simulink model "CrazyClover_trajectory_tracking"  (R2020b)
settings: Solver=VariableStepAuto  StartTime=0.0  StopTime=30  RelTol=1e-3
values from neighbouring files (symbols this model uses):
  controller_matrix = [mass/(4*gravity)*1000 mass/(4*gravity)*1000 mass/(4*gravity)*1000 mass/(4*gravity)*1000 ... (first row only)    [sim_param.m]
  kM1 = Armlength /sqrt(2)    [sim_param.m]
  kM2 = Armlength /sqrt(2)    [sim_param.m]
  kM3 = 1    [sim_param.m]
undefined symbols (not defined in the file or in its folder): Pitchrate, Rollrate, traj, Yawrate
libraries: pid_lib x6
settings Model: Creator=kt012  LastModifiedBy=kt012

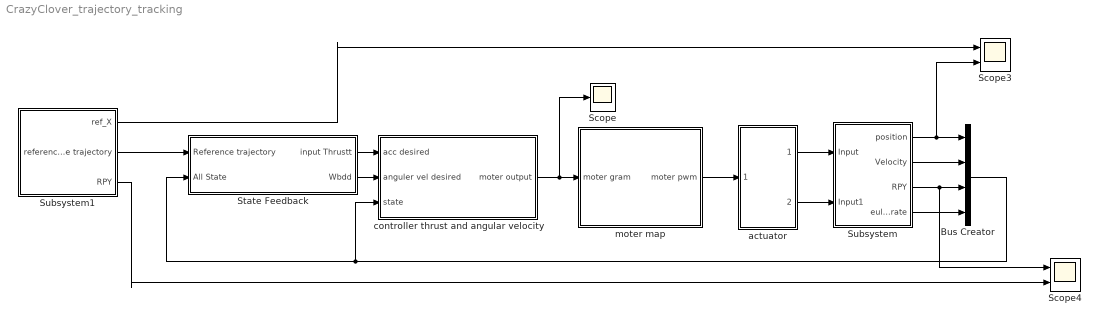
== system CrazyClover_trajectory_tracking ==
  Bus Creator : BusCreator  Inputs=4
  Scope : Scope
  Scope3 : Scope  NumInputPorts=2
  Scope4 : Scope  NumInputPorts=2
  State Feedback : Subsystem
  Subsystem : Subsystem
  Subsystem1 : Subsystem
  actuator : Subsystem
  controller thrust and angular velocity : Subsystem
  moter map : Subsystem
  wires:
  actuator/1(Input) -> Subsystem/1(Input)
  State Feedback/2("Wbdd ") -> controller thrust and angular velocity/2(anguler vel desired)
  actuator/2(Input1) -> Subsystem/2(Input1)
  Subsystem/1(position) -> Scope3/2, Bus Creator/1
  controller thrust and angular velocity/1(moter output) -> Scope/1, moter map/1(moter gram)
  State Feedback/1(input Thrustt) -> controller thrust and angular velocity/1(acc desired)
  moter map/1(moter pwm) -> actuator/1(PWM)
  Subsystem/3(RPY) -> Scope4/1, Bus Creator/3
  Subsystem/4(euler rate) -> Bus Creator/4
  Subsystem/2(Velocity) -> Bus Creator/2
  Bus Creator/1 -> controller thrust and angular velocity/3(state), State Feedback/2(All State)
  Subsystem1/1(ref_X) -> Scope3/1
  Subsystem1/2(reference trajectory) -> State Feedback/1(Reference trajectory)
  Subsystem1/3(RPY) -> Scope4/2

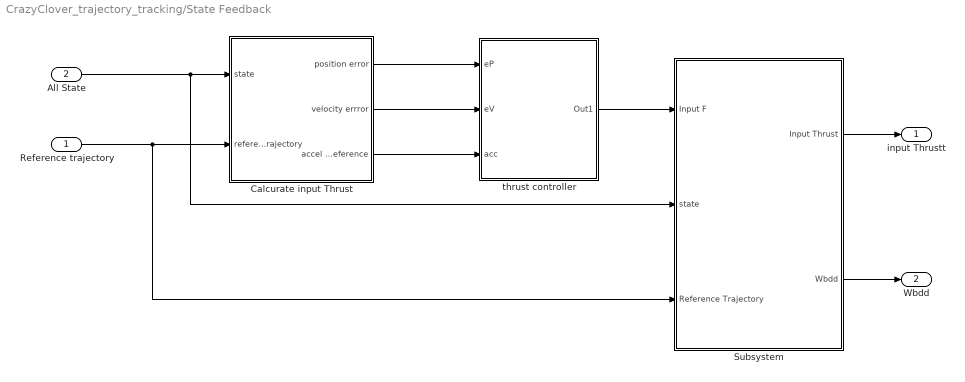
== system CrazyClover_trajectory_tracking/State Feedback ==
  Reference trajectory : Inport
  All State : Inport  Port=2
  Calcurate input Thrust : Subsystem
  Subsystem : Subsystem
  thrust controller : Subsystem
  input Thrustt : Outport
  "Wbdd " : Outport  Port=2  VectorParamsAs1DForOutWhenUnconnected=off
  wires:
  All State/1 -> Calcurate input Thrust/1(state), Subsystem/2(state)
  Reference trajectory/1 -> Calcurate input Thrust/2(reference trajectory), Subsystem/3(Reference Trajectory)
  Subsystem/2("Wbdd ") -> "Wbdd "/1
  Subsystem/1(Input Thrust) -> input Thrustt/1
  Calcurate input Thrust/1(position error) -> thrust controller/1(eP)
  Calcurate input Thrust/2(velocity errror) -> thrust controller/2(eV)
  Calcurate input Thrust/3(accel reference) -> thrust controller/3(acc)
  thrust controller/1(Out1) -> Subsystem/1(Input F)

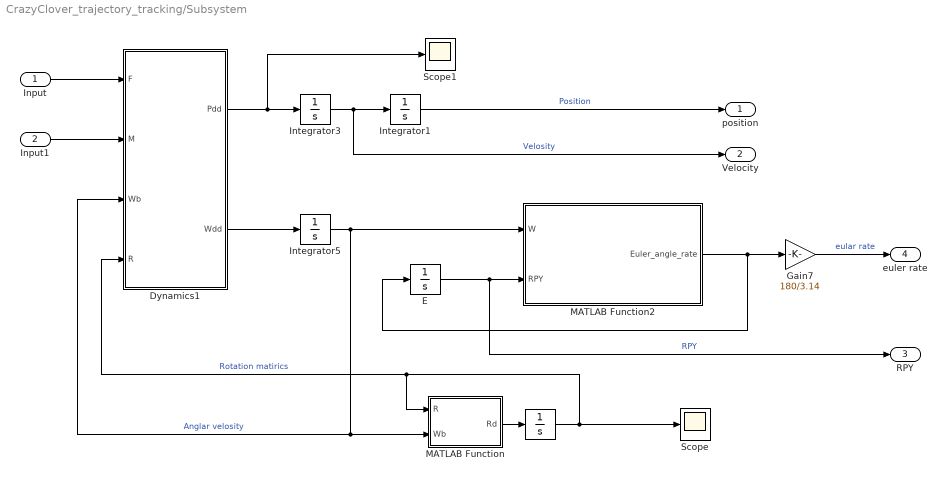
== system CrazyClover_trajectory_tracking/Subsystem ==
  Input : Inport
  Input1 : Inport  Port=2
  " " : Integrator  InitialCondition=[1 0 0; 0 1 0; 0 0 1];  ContinuousStateAttributes="\"\""
  Dynamics1 : MATLAB Function  TreatAsAtomicUnit=on
  E : Integrator  InitialCondition=[0 0 0];
  Gain7 : Gain  Gain=180/3.14
  Integrator1 : Integrator  InitialCondition=[0 0 0];
  Integrator3 : Integrator  InitialCondition=[0 0 0];
  Integrator5 : Integrator  InitialCondition=[0 0 0];
  MATLAB Function : MATLAB Function  TreatAsAtomicUnit=on
  MATLAB Function2 : MATLAB Function  TreatAsAtomicUnit=on
  Scope : Scope
  Scope1 : Scope
  position : Outport
  Velocity : Outport  Port=2
  RPY : Outport  Port=3
  euler rate : Outport  Port=4
  wires:
  MATLAB Function2/1(Euler_angle_rate) -> E/1, Gain7/1
  Dynamics1/1(Pdd) -> Integrator3/1, Scope1/1
  Integrator1/1 -> position/1  "Position"
  Integrator3/1 -> Velocity/1, Integrator1/1  "Velosity"
  E/1 -> RPY/1, MATLAB Function2/2(RPY)  "RPY"
  Dynamics1/2(Wdd) -> Integrator5/1
  Gain7/1 -> euler rate/1  "eular rate"
  MATLAB Function/1(Rd) -> " "/1
  Integrator5/1 -> MATLAB Function/2(Wb), Dynamics1/3(Wb), MATLAB Function2/1(W)  "Anglar velosity"
  " "/1 -> Dynamics1/4(R), MATLAB Function/1(R), Scope/1  "Rotation matirics"
  Input1/1 -> Dynamics1/2(M)
  Input/1 -> Dynamics1/1(F)

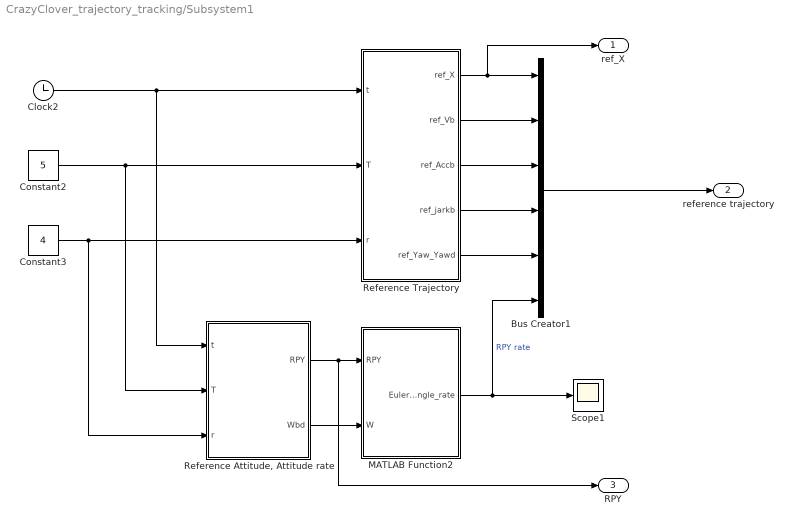
== system CrazyClover_trajectory_tracking/Subsystem1 ==
  Bus Creator1 : BusCreator  Inputs=6
  Clock2 : Clock
  Constant2 : Constant  Value=5
  Constant3 : Constant  Value=4
  MATLAB Function2 : MATLAB Function  TreatAsAtomicUnit=on
  "Reference Attitude, Attitude rate " : MATLAB Function  TreatAsAtomicUnit=on
  Reference Trajectory : MATLAB Function  TreatAsAtomicUnit=on
  Scope1 : Scope
  ref_X : Outport
  reference trajectory : Outport  Port=2
  RPY : Outport  Port=3
  wires:
  Reference Trajectory/1(ref_X) -> ref_X/1, Bus Creator1/1
  Reference Trajectory/4(ref_jarkb) -> Bus Creator1/4
  Reference Trajectory/3(ref_Accb) -> Bus Creator1/3
  MATLAB Function2/1(Euler_angle_rate) -> Bus Creator1/6, Scope1/1  "RPY rate"
  Constant3/1 -> "Reference Attitude, Attitude rate "/3(r), Reference Trajectory/3(r)
  Reference Trajectory/5(ref_Yaw_Yawd) -> Bus Creator1/5
  Clock2/1 -> "Reference Attitude, Attitude rate "/1(t), Reference Trajectory/1(t)
  Constant2/1 -> "Reference Attitude, Attitude rate "/2(T), Reference Trajectory/2(T)
  "Reference Attitude, Attitude rate "/2(Wbd) -> MATLAB Function2/2(W)
  Reference Trajectory/2(ref_Vb) -> Bus Creator1/2
  Bus Creator1/1 -> reference trajectory/1
  "Reference Attitude, Attitude rate "/1(RPY) -> RPY/1, MATLAB Function2/1(RPY)

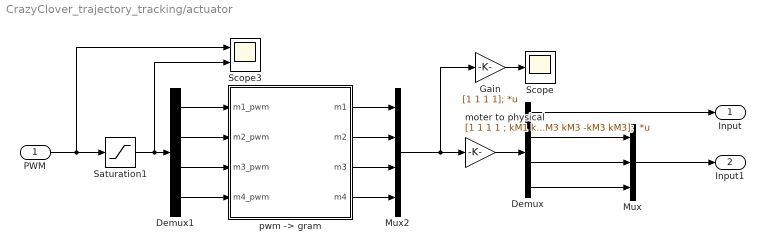
== system CrazyClover_trajectory_tracking/actuator ==
  PWM : Inport
  Demux : Demux
  Demux1 : Demux
  Gain : Gain  Gain=[1 1 1 1];  Multiplication=Matrix(K*u)
  Mux : Mux  Inputs=3
  Mux2 : Mux
  Saturation1 : Saturate  UpperLimit=40000  LowerLimit=0
  Scope : Scope
  Scope3 : Scope  NumInputPorts=2
  moter to physical : Gain  Gain=[1 1 1 1 ; kM1 kM1 -kM1 -kM1; -kM2 kM2 kM2 -kM2; -kM3 kM3 -kM3 kM3];  Multiplication=Matrix(K*u)
  "pwm -> gram" : MATLAB Function  TreatAsAtomicUnit=on
  Input : Outport
  Input1 : Outport  Port=2
  wires:
  Demux/2 -> Mux/1
  "pwm -> gram"/3(m3) -> Mux2/3
  Demux1/2 -> "pwm -> gram"/2(m2_pwm)
  Demux/4 -> Mux/3
  Demux/3 -> Mux/2
  moter to physical/1 -> Demux/1
  "pwm -> gram"/1(m1) -> Mux2/1
  Mux2/1 -> Gain/1, moter to physical/1
  Gain/1 -> Scope/1
  Saturation1/1 -> Scope3/2, Demux1/1
  PWM/1 -> Scope3/1, Saturation1/1
  Demux1/3 -> "pwm -> gram"/3(m3_pwm)
  "pwm -> gram"/4(m4) -> Mux2/4
  "pwm -> gram"/2(m2) -> Mux2/2
  Demux1/4 -> "pwm -> gram"/4(m4_pwm)
  Demux1/1 -> "pwm -> gram"/1(m1_pwm)
  Mux/1 -> Input1/1
  Demux/1 -> Input/1

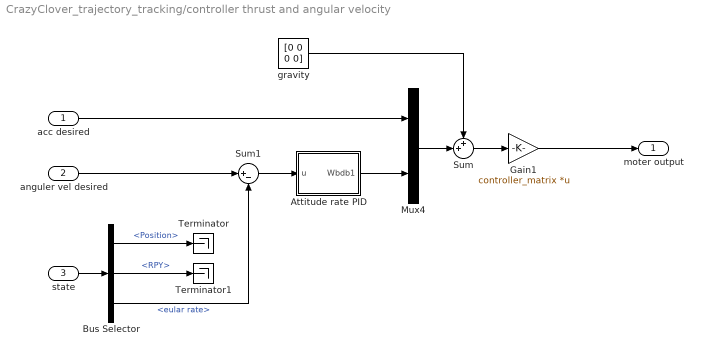
== system CrazyClover_trajectory_tracking/controller thrust and angular velocity ==
  acc desired : Inport
  anguler vel desired : Inport  Port=2
  state : Inport  Port=3
  Attitude rate PID : Subsystem
  Bus Selector : BusSelector  OutputSignals=Position,RPY,eular rate
  Gain1 : Gain  Gain=controller_matrix  Multiplication=Matrix(K*u)
  Mux4 : Mux  Inputs=2
  Sum : Sum  Inputs=++|
  Sum1 : Sum  Inputs=|+-
  Terminator : Terminator
  Terminator1 : Terminator
  gravity : Constant  Value=[0 0 0 0]
  moter output : Outport
  wires:
  Sum/1 -> Gain1/1
  Gain1/1 -> moter output/1
  Mux4/1 -> Sum/2
  gravity/1 -> Sum/1
  Attitude rate PID/1(Wbdb1) -> Mux4/2
  state/1 -> Bus Selector/1
  Bus Selector/3 -> Sum1/2  "<eular rate>"
  Sum1/1 -> Attitude rate PID/1(u)
  Bus Selector/1 -> Terminator/1  "<Position>"
  Bus Selector/2 -> Terminator1/1  "<RPY>"
  anguler vel desired/1 -> Sum1/1
  acc desired/1 -> Mux4/1

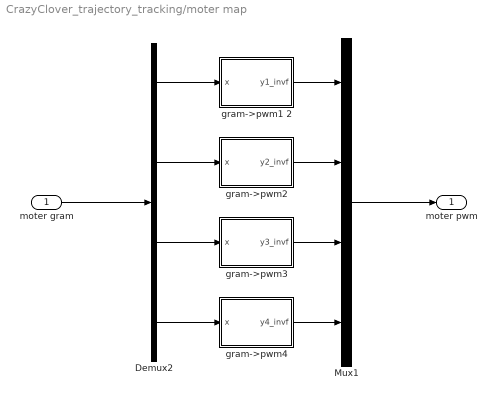
== system CrazyClover_trajectory_tracking/moter map ==
  moter gram : Inport
  Demux2 : Demux
  Mux1 : Mux
  gram->pwm1 2 : MATLAB Function  TreatAsAtomicUnit=on
  gram->pwm2 : MATLAB Function  TreatAsAtomicUnit=on
  gram->pwm3 : MATLAB Function  TreatAsAtomicUnit=on
  gram->pwm4 : MATLAB Function  TreatAsAtomicUnit=on
  moter pwm : Outport
  wires:
  Demux2/4 -> gram->pwm4/1(x)
  Demux2/3 -> gram->pwm3/1(x)
  gram->pwm4/1(y4_invf) -> Mux1/4
  Demux2/2 -> gram->pwm2/1(x)
  gram->pwm3/1(y3_invf) -> Mux1/3
  gram->pwm2/1(y2_invf) -> Mux1/2
  gram->pwm1 2/1(y1_invf) -> Mux1/1
  Demux2/1 -> gram->pwm1 2/1(x)
  Mux1/1 -> moter pwm/1
  moter gram/1 -> Demux2/1

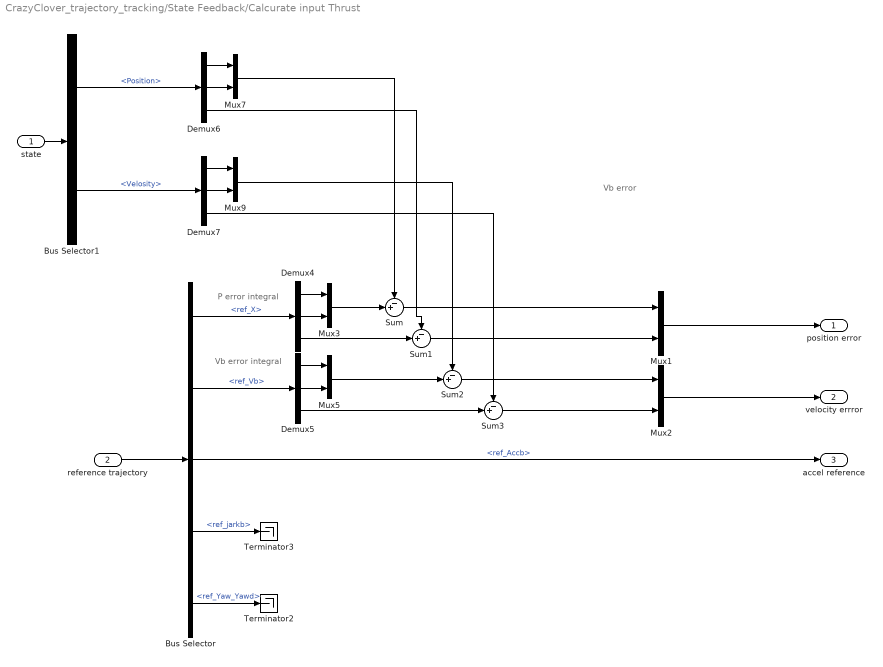
== system CrazyClover_trajectory_tracking/State Feedback/Calcurate input Thrust ==
  note: P error integral
  note: Vb error
  note: Vb error integral
  state : Inport
  reference trajectory : Inport  Port=2
  Bus Selector : BusSelector  OutputSignals=ref_X,ref_Vb,ref_Accb,ref_jarkb,ref_Yaw_Yawd
  Bus Selector1 : BusSelector  OutputSignals=Position,Velosity
  Demux{4..7} (4 alike) : Demux  Outputs=3
  Mux{1..3,5,7,9} (6 alike) : Mux  Inputs=2
  Sum{,1..3} (4 alike) : Sum  Inputs=-+|
  Terminator2 : Terminator
  Terminator3 : Terminator
  position error : Outport
  velocity errror : Outport  Port=2
  accel reference : Outport  Port=3
  wires:
  Demux6/2 -> Mux7/2
  Demux5/3 -> Sum3/2
  Bus Selector/1 -> Demux4/1  "<ref_X>"
  reference trajectory/1 -> Bus Selector/1
  Mux5/1 -> Sum2/2
  Bus Selector/5 -> Terminator2/1  "<ref_Yaw_Yawd>"
  Sum3/1 -> Mux2/2
  Bus Selector/4 -> Terminator3/1  "<ref_jarkb>"
  Mux2/1 -> velocity errror/1
  Demux4/1 -> Mux3/1
  Bus Selector/3 -> accel reference/1  "<ref_Accb>"
  state/1 -> Bus Selector1/1
  Demux4/3 -> Sum1/2
  Sum2/1 -> Mux2/1
  Bus Selector1/1 -> Demux6/1  "<Position>"
  Demux6/1 -> Mux7/1
  Demux7/3 -> Sum3/1
  Mux1/1 -> position error/1
  Mux7/1 -> Sum/1
  Mux9/1 -> Sum2/1
  Sum1/1 -> Mux1/2
  Bus Selector1/2 -> Demux7/1  "<Velosity>"
  Demux4/2 -> Mux3/2
  Demux5/2 -> Mux5/2
  Sum/1 -> Mux1/1
  Demux7/1 -> Mux9/1
  Bus Selector/2 -> Demux5/1  "<ref_Vb>"
  Demux7/2 -> Mux9/2
  Demux6/3 -> Sum1/1
  Demux5/1 -> Mux5/1
  Mux3/1 -> Sum/2

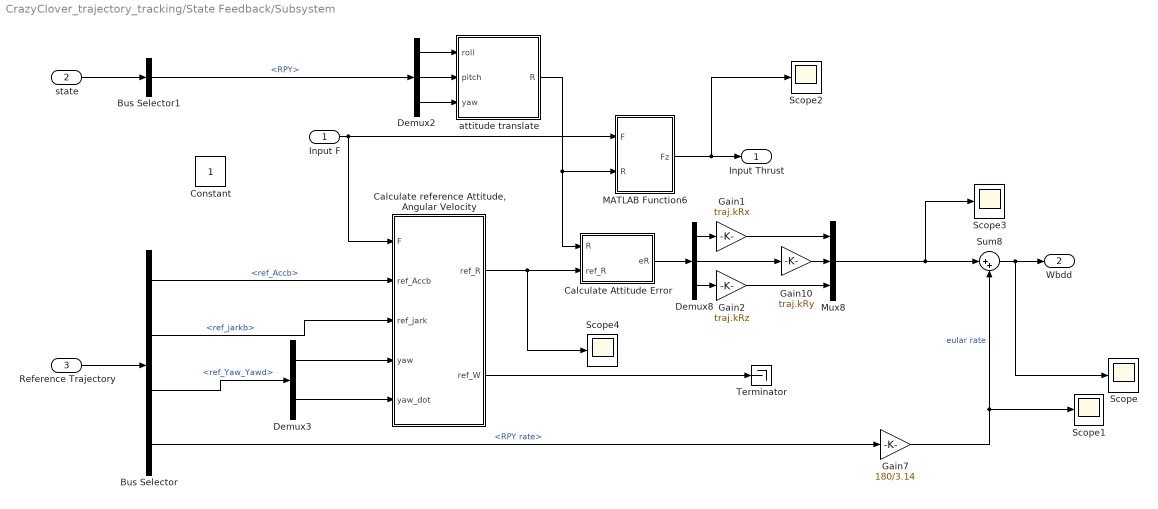
== system CrazyClover_trajectory_tracking/State Feedback/Subsystem ==
  Input F : Inport
  state : Inport  Port=2
  Reference Trajectory : Inport  Port=3
  Bus Selector : BusSelector  OutputSignals=ref_Accb,ref_jarkb,ref_Yaw_Yawd,RPY rate
  Bus Selector1 : BusSelector  OutputSignals=RPY
  Calculate Attitude Error : MATLAB Function  TreatAsAtomicUnit=on
  "Calculate reference Attitude, Angular Velocity" : MATLAB Function  TreatAsAtomicUnit=on
  Constant : Constant
  Demux2 : Demux  Outputs=3
  Demux3 : Demux  Outputs=2
  Demux8 : Demux  Outputs=3
  Gain1 : Gain  Gain=traj.kRx
  Gain10 : Gain  Gain=traj.kRy
  Gain2 : Gain  Gain=traj.kRz
  Gain7 : Gain  Gain=180/3.14
  MATLAB Function6 : MATLAB Function
  Mux8 : Mux  Inputs=3
  Scope{,1..4} (5 alike) : Scope
  Sum8 : Sum  Inputs=|++
  Terminator : Terminator
  attitude translate : MATLAB Function  TreatAsAtomicUnit=on
  Input Thrust : Outport
  "Wbdd " : Outport  Port=2  VectorParamsAs1DForOutWhenUnconnected=off
  wires:
  Demux8/3 -> Gain2/1
  "Calculate reference Attitude, Angular Velocity"/1(ref_R) -> Scope4/1, Calculate Attitude Error/2(ref_R)
  Sum8/1 -> Scope/1, "Wbdd "/1
  Input F/1 -> "Calculate reference Attitude, Angular Velocity"/1(F), MATLAB Function6/1(F)
  Demux8/2 -> Gain10/1
  attitude translate/1(R) -> Calculate Attitude Error/1(R), MATLAB Function6/2(R)
  Demux8/1 -> Gain1/1
  Gain10/1 -> Mux8/2
  Bus Selector1/1 -> Demux2/1  "<RPY>"
  Bus Selector/3 -> Demux3/1  "<ref_Yaw_Yawd>"
  Reference Trajectory/1 -> Bus Selector/1
  Bus Selector/1 -> "Calculate reference Attitude, Angular Velocity"/2(ref_Accb)  "<ref_Accb>"
  Demux3/1 -> "Calculate reference Attitude, Angular Velocity"/4(yaw)
  Demux3/2 -> "Calculate reference Attitude, Angular Velocity"/5(yaw_dot)
  state/1 -> Bus Selector1/1
  MATLAB Function6/1(Fz) -> Scope2/1, Input Thrust/1
  Bus Selector/2 -> "Calculate reference Attitude, Angular Velocity"/3(ref_jark)  "<ref_jarkb>"
  Demux2/1 -> attitude translate/1(roll)
  Demux2/2 -> attitude translate/2(pitch)
  Demux2/3 -> attitude translate/3(yaw)
  Calculate Attitude Error/1(eR) -> Demux8/1
  "Calculate reference Attitude, Angular Velocity"/2(ref_W) -> Terminator/1
  Bus Selector/4 -> Gain7/1  "<RPY rate>"
  Mux8/1 -> Scope3/1, Sum8/1
  Gain1/1 -> Mux8/1
  Gain2/1 -> Mux8/3
  Gain7/1 -> Sum8/2, Scope1/1  "eular rate"

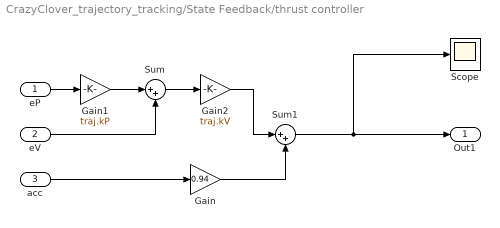
== system CrazyClover_trajectory_tracking/State Feedback/thrust controller ==
  eP : Inport
  eV : Inport  Port=2
  acc : Inport  Port=3
  Gain : Gain  Gain=0.94
  Gain1 : Gain  Gain=traj.kP
  Gain2 : Gain  Gain=traj.kV
  Scope : Scope
  Sum : Sum  Inputs=|++
  Sum1 : Sum  Inputs=|++
  Out1 : Outport
  wires:
  acc/1 -> Gain/1
  Sum/1 -> Gain2/1
  Sum1/1 -> Scope/1, Out1/1
  eP/1 -> Gain1/1
  eV/1 -> Sum/2
  Gain1/1 -> Sum/1
  Gain2/1 -> Sum1/1
  Gain/1 -> Sum1/2

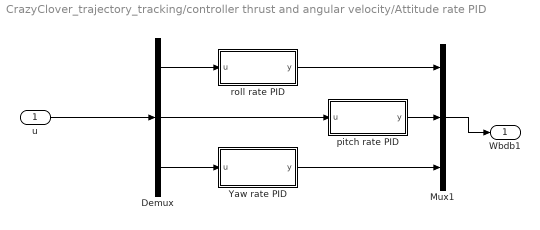
== system CrazyClover_trajectory_tracking/controller thrust and angular velocity/Attitude rate PID ==
  u : Inport
  Demux : Demux  Outputs=3
  Mux1 : Mux  Inputs=3
  "Yaw rate PID " : Subsystem
  pitch rate PID : Subsystem
  "roll rate PID " : Subsystem
  Wbdb1 : Outport
  wires:
  "roll rate PID "/1(y) -> Mux1/1
  pitch rate PID/1(y) -> Mux1/2
  Demux/2 -> pitch rate PID/1(u)
  u/1 -> Demux/1
  Demux/3 -> "Yaw rate PID "/1(u)
  Demux/1 -> "roll rate PID "/1(u)
  "Yaw rate PID "/1(y) -> Mux1/3
  Mux1/1 -> Wbdb1/1

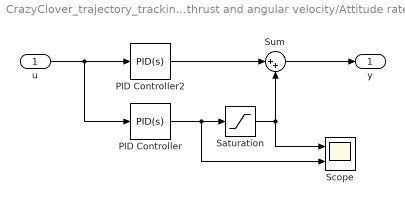
== system CrazyClover_trajectory_tracking/controller thrust and angular velocity/Attitude rate PID/Yaw rate PID  ==
  u : Inport
  PID Controller : pid_lib/PID Controller  Controller=PID  Form=Parallel  TimeDomain=Continuous-time  UseExternalTs=off  SampleTime=-1  IntegratorMethod=Forward Euler  FilterMethod=Forward Euler  ControllerParametersSource=internal  P=0  I=Yawrate.ki  D=0  UseFilter=on  N=100  TunerSelectOption=Transfer Function Based (PID Tuner App)  InitialConditionSource=internal  InitialConditionForIntegrator=0  InitialConditionForFilter=0  DifferentiatorICPrevScaledInput=0  ExternalReset=none  TrackingMode=off  Kt=1  LimitOutput=off  SatLimitsSource=internal  UpperSaturationLimit=inf  LowerSaturationLimit=-inf  LinearizeAsGain=on  AntiWindupMode=none  Kb=1  POutMin=[]  POutMax=[]  IOutMin=[]  IOutMax=[]  DOutMin=[]  DOutMax=[]  NOutMin=[]  NOutMax=[]  SumOutMin=[]  SumOutMax=[]  SaturationOutMin=[]  SaturationOutMax=[]  PParamMin=[]  PParamMax=[]  IParamMin=[]  IParamMax=[]  DParamMin=[]  DParamMax=[]  NParamMin=[]  NParamMax=[]  KbParamMin=[]  KbParamMax=[]  KtParamMin=[]  KtParamMax=[]  KbOutMin=[]  KbOutMax=[]  KtOutMin=[]  KtOutMax=[]  IntegratorOutMin=[]  IntegratorOutMax=[]  FilterOutMin=[]  FilterOutMax=[]  SumI1OutMin=[]  SumI1OutMax=[]  SumI2OutMin=[]  SumI2OutMax=[]  SumI3OutMin=[]  SumI3OutMax=[]  SumI4OutMin=[]  SumI4OutMax=[]  SumDOutMin=[]  SumDOutMax=[]  DifferentiatorOutMin=[]  DifferentiatorOutMax=[]  FilterDiffOutCoefMin=[]  FilterDiffOutCoefMax=[]  ReciprocalOutMin=[]  ReciprocalOutMax=[]  SumDenOutMin=[]  SumDenOutMax=[]  SumNumOutMin=[]  SumNumOutMax=[]  DivideOutMin=[]  DivideOutMax=[]  UdiffTsProdOutMin=[]  UdiffTsProdOutMax=[]  NTsProdOutMin=[]  NTsProdOutMax=[]  UintegralTsProdOutMin=[]  UintegralTsProdOutMax=[]  UngainTsProdOutMin=[]  UngainTsProdOutMax=[]  IntegratorContinuousStateAttributes=''  IntegratorStateMustResolveToSignalObject=off  IntegratorRTWStateStorageClass=Auto  FilterContinuousStateAttributes=''  FilterStateMustResolveToSignalObject=off  FilterRTWStateStorageClass=Auto  ParallelPVariant=InternalParameters  IdealPVariant=Disabled  IVariant=InternalParameters  DVariant=InternalParameters  IntegratorVariant=Continuous  SatVariant=Disabled  AWVariant=Passthrough  PCopyVariant=Disabled  TRVariant=Disabled  FdbkBlocksVariant=Forward  IdealPFdbkVariant=Disabled  SatFdbkVariant=Disabled  DerivativeFilterVariant=ContFilter  NVariant=InternalParameters  NCopyVariant=Disabled  FilterICVariant=InternalICsFilter  IntegratorICVariant=InternalICs  ExternalResetVariant=Disabled  TRSumVariant=Passthrough  SumFdbkVariant=Disabled  SumVariant=Sum_PID  TsampFilterVariant=InternalTs  TsampNgainVariant=Passthrough  TsampIntegralVariant=Passthrough  ExternalSaturationOutDataTypeStr=Inherit: Same as second input
  PID Controller2 : pid_lib/PID Controller  Controller=PID  Form=Parallel  TimeDomain=Continuous-time  UseExternalTs=off  SampleTime=-1  IntegratorMethod=Forward Euler  FilterMethod=Forward Euler  ControllerParametersSource=internal  P=Yawrate.kp  I=0  D=0  UseFilter=on  N=100  TunerSelectOption=Transfer Function Based (PID Tuner App)  InitialConditionSource=internal  InitialConditionForIntegrator=0  InitialConditionForFilter=0  DifferentiatorICPrevScaledInput=0  ExternalReset=none  TrackingMode=off  Kt=1  LimitOutput=off  SatLimitsSource=internal  UpperSaturationLimit=inf  LowerSaturationLimit=-inf  LinearizeAsGain=on  AntiWindupMode=none  Kb=1  POutMin=[]  POutMax=[]  IOutMin=[]  IOutMax=[]  DOutMin=[]  DOutMax=[]  NOutMin=[]  NOutMax=[]  SumOutMin=[]  SumOutMax=[]  SaturationOutMin=[]  SaturationOutMax=[]  PParamMin=[]  PParamMax=[]  IParamMin=[]  IParamMax=[]  DParamMin=[]  DParamMax=[]  NParamMin=[]  NParamMax=[]  KbParamMin=[]  KbParamMax=[]  KtParamMin=[]  KtParamMax=[]  KbOutMin=[]  KbOutMax=[]  KtOutMin=[]  KtOutMax=[]  IntegratorOutMin=[]  IntegratorOutMax=[]  FilterOutMin=[]  FilterOutMax=[]  SumI1OutMin=[]  SumI1OutMax=[]  SumI2OutMin=[]  SumI2OutMax=[]  SumI3OutMin=[]  SumI3OutMax=[]  SumI4OutMin=[]  SumI4OutMax=[]  SumDOutMin=[]  SumDOutMax=[]  DifferentiatorOutMin=[]  DifferentiatorOutMax=[]  FilterDiffOutCoefMin=[]  FilterDiffOutCoefMax=[]  ReciprocalOutMin=[]  ReciprocalOutMax=[]  SumDenOutMin=[]  SumDenOutMax=[]  SumNumOutMin=[]  SumNumOutMax=[]  DivideOutMin=[]  DivideOutMax=[]  UdiffTsProdOutMin=[]  UdiffTsProdOutMax=[]  NTsProdOutMin=[]  NTsProdOutMax=[]  UintegralTsProdOutMin=[]  UintegralTsProdOutMax=[]  UngainTsProdOutMin=[]  UngainTsProdOutMax=[]  IntegratorContinuousStateAttributes=''  IntegratorStateMustResolveToSignalObject=off  IntegratorRTWStateStorageClass=Auto  FilterContinuousStateAttributes=''  FilterStateMustResolveToSignalObject=off  FilterRTWStateStorageClass=Auto  ParallelPVariant=InternalParameters  IdealPVariant=Disabled  IVariant=InternalParameters  DVariant=InternalParameters  IntegratorVariant=Continuous  SatVariant=Disabled  AWVariant=Passthrough  PCopyVariant=Disabled  TRVariant=Disabled  FdbkBlocksVariant=Forward  IdealPFdbkVariant=Disabled  SatFdbkVariant=Disabled  DerivativeFilterVariant=ContFilter  NVariant=InternalParameters  NCopyVariant=Disabled  FilterICVariant=InternalICsFilter  IntegratorICVariant=InternalICs  ExternalResetVariant=Disabled  TRSumVariant=Passthrough  SumFdbkVariant=Disabled  SumVariant=Sum_PID  TsampFilterVariant=InternalTs  TsampNgainVariant=Passthrough  TsampIntegralVariant=Passthrough  ExternalSaturationOutDataTypeStr=Inherit: Same as second input
  Saturation : Saturate  UpperLimit=Yawrate.intupper  LowerLimit=Yawrate.intlower
  Scope : Scope  NumInputPorts=2
  Sum : Sum  Inputs=|++
  y : Outport
  wires:
  PID Controller2/1 -> Sum/1
  u/1 -> PID Controller/1, PID Controller2/1
  Sum/1 -> y/1
  PID Controller/1 -> Scope/2, Saturation/1
  Saturation/1 -> Sum/2, Scope/1

== system CrazyClover_trajectory_tracking/controller thrust and angular velocity/Attitude rate PID/pitch rate PID ==
  u : Inport
  PID Controller1 : pid_lib/PID Controller  Controller=PID  Form=Parallel  TimeDomain=Continuous-time  UseExternalTs=off  SampleTime=-1  IntegratorMethod=Forward Euler  FilterMethod=Forward Euler  ControllerParametersSource=internal  P=0  I=Pitchrate.ki  D=0  UseFilter=on  N=100  TunerSelectOption=Transfer Function Based (PID Tuner App)  InitialConditionSource=internal  InitialConditionForIntegrator=0  InitialConditionForFilter=0  DifferentiatorICPrevScaledInput=0  ExternalReset=none  TrackingMode=off  Kt=1  LimitOutput=off  SatLimitsSource=internal  UpperSaturationLimit=inf  LowerSaturationLimit=-inf  LinearizeAsGain=on  AntiWindupMode=none  Kb=1  POutMin=[]  POutMax=[]  IOutMin=[]  IOutMax=[]  DOutMin=[]  DOutMax=[]  NOutMin=[]  NOutMax=[]  SumOutMin=[]  SumOutMax=[]  SaturationOutMin=[]  SaturationOutMax=[]  PParamMin=[]  PParamMax=[]  IParamMin=[]  IParamMax=[]  DParamMin=[]  DParamMax=[]  NParamMin=[]  NParamMax=[]  KbParamMin=[]  KbParamMax=[]  KtParamMin=[]  KtParamMax=[]  KbOutMin=[]  KbOutMax=[]  KtOutMin=[]  KtOutMax=[]  IntegratorOutMin=[]  IntegratorOutMax=[]  FilterOutMin=[]  FilterOutMax=[]  SumI1OutMin=[]  SumI1OutMax=[]  SumI2OutMin=[]  SumI2OutMax=[]  SumI3OutMin=[]  SumI3OutMax=[]  SumI4OutMin=[]  SumI4OutMax=[]  SumDOutMin=[]  SumDOutMax=[]  DifferentiatorOutMin=[]  DifferentiatorOutMax=[]  FilterDiffOutCoefMin=[]  FilterDiffOutCoefMax=[]  ReciprocalOutMin=[]  ReciprocalOutMax=[]  SumDenOutMin=[]  SumDenOutMax=[]  SumNumOutMin=[]  SumNumOutMax=[]  DivideOutMin=[]  DivideOutMax=[]  UdiffTsProdOutMin=[]  UdiffTsProdOutMax=[]  NTsProdOutMin=[]  NTsProdOutMax=[]  UintegralTsProdOutMin=[]  UintegralTsProdOutMax=[]  UngainTsProdOutMin=[]  UngainTsProdOutMax=[]  IntegratorContinuousStateAttributes=''  IntegratorStateMustResolveToSignalObject=off  IntegratorRTWStateStorageClass=Auto  FilterContinuousStateAttributes=''  FilterStateMustResolveToSignalObject=off  FilterRTWStateStorageClass=Auto  ParallelPVariant=InternalParameters  IdealPVariant=Disabled  IVariant=InternalParameters  DVariant=InternalParameters  IntegratorVariant=Continuous  SatVariant=Disabled  AWVariant=Passthrough  PCopyVariant=Disabled  TRVariant=Disabled  FdbkBlocksVariant=Forward  IdealPFdbkVariant=Disabled  SatFdbkVariant=Disabled  DerivativeFilterVariant=ContFilter  NVariant=InternalParameters  NCopyVariant=Disabled  FilterICVariant=InternalICsFilter  IntegratorICVariant=InternalICs  ExternalResetVariant=Disabled  TRSumVariant=Passthrough  SumFdbkVariant=Disabled  SumVariant=Sum_PID  TsampFilterVariant=InternalTs  TsampNgainVariant=Passthrough  TsampIntegralVariant=Passthrough  ExternalSaturationOutDataTypeStr=Inherit: Same as second input
  PID Controller2 : pid_lib/PID Controller  Controller=PID  Form=Parallel  TimeDomain=Continuous-time  UseExternalTs=off  SampleTime=-1  IntegratorMethod=Forward Euler  FilterMethod=Forward Euler  ControllerParametersSource=internal  P=Pitchrate.kp  I=0  D=0  UseFilter=on  N=100  TunerSelectOption=Transfer Function Based (PID Tuner App)  InitialConditionSource=internal  InitialConditionForIntegrator=0  InitialConditionForFilter=0  DifferentiatorICPrevScaledInput=0  ExternalReset=none  TrackingMode=off  Kt=1  LimitOutput=off  SatLimitsSource=internal  UpperSaturationLimit=inf  LowerSaturationLimit=-inf  LinearizeAsGain=on  AntiWindupMode=none  Kb=1  POutMin=[]  POutMax=[]  IOutMin=[]  IOutMax=[]  DOutMin=[]  DOutMax=[]  NOutMin=[]  NOutMax=[]  SumOutMin=[]  SumOutMax=[]  SaturationOutMin=[]  SaturationOutMax=[]  PParamMin=[]  PParamMax=[]  IParamMin=[]  IParamMax=[]  DParamMin=[]  DParamMax=[]  NParamMin=[]  NParamMax=[]  KbParamMin=[]  KbParamMax=[]  KtParamMin=[]  KtParamMax=[]  KbOutMin=[]  KbOutMax=[]  KtOutMin=[]  KtOutMax=[]  IntegratorOutMin=[]  IntegratorOutMax=[]  FilterOutMin=[]  FilterOutMax=[]  SumI1OutMin=[]  SumI1OutMax=[]  SumI2OutMin=[]  SumI2OutMax=[]  SumI3OutMin=[]  SumI3OutMax=[]  SumI4OutMin=[]  SumI4OutMax=[]  SumDOutMin=[]  SumDOutMax=[]  DifferentiatorOutMin=[]  DifferentiatorOutMax=[]  FilterDiffOutCoefMin=[]  FilterDiffOutCoefMax=[]  ReciprocalOutMin=[]  ReciprocalOutMax=[]  SumDenOutMin=[]  SumDenOutMax=[]  SumNumOutMin=[]  SumNumOutMax=[]  DivideOutMin=[]  DivideOutMax=[]  UdiffTsProdOutMin=[]  UdiffTsProdOutMax=[]  NTsProdOutMin=[]  NTsProdOutMax=[]  UintegralTsProdOutMin=[]  UintegralTsProdOutMax=[]  UngainTsProdOutMin=[]  UngainTsProdOutMax=[]  IntegratorContinuousStateAttributes=''  IntegratorStateMustResolveToSignalObject=off  IntegratorRTWStateStorageClass=Auto  FilterContinuousStateAttributes=''  FilterStateMustResolveToSignalObject=off  FilterRTWStateStorageClass=Auto  ParallelPVariant=InternalParameters  IdealPVariant=Disabled  IVariant=InternalParameters  DVariant=InternalParameters  IntegratorVariant=Continuous  SatVariant=Disabled  AWVariant=Passthrough  PCopyVariant=Disabled  TRVariant=Disabled  FdbkBlocksVariant=Forward  IdealPFdbkVariant=Disabled  SatFdbkVariant=Disabled  DerivativeFilterVariant=ContFilter  NVariant=InternalParameters  NCopyVariant=Disabled  FilterICVariant=InternalICsFilter  IntegratorICVariant=InternalICs  ExternalResetVariant=Disabled  TRSumVariant=Passthrough  SumFdbkVariant=Disabled  SumVariant=Sum_PID  TsampFilterVariant=InternalTs  TsampNgainVariant=Passthrough  TsampIntegralVariant=Passthrough  ExternalSaturationOutDataTypeStr=Inherit: Same as second input
  Saturation : Saturate  UpperLimit=Pitchrate.intupper  LowerLimit=Pitchrate.intlower
  Scope : Scope  NumInputPorts=2
  Sum : Sum  Inputs=|++
  y : Outport
  wires:
  PID Controller2/1 -> Sum/1
  u/1 -> PID Controller1/1, PID Controller2/1
  Sum/1 -> y/1
  PID Controller1/1 -> Scope/2, Saturation/1
  Saturation/1 -> Sum/2, Scope/1

== system CrazyClover_trajectory_tracking/controller thrust and angular velocity/Attitude rate PID/roll rate PID  ==
  u : Inport
  PID Controller1 : pid_lib/PID Controller  Controller=PID  Form=Parallel  TimeDomain=Continuous-time  UseExternalTs=off  SampleTime=-1  IntegratorMethod=Forward Euler  FilterMethod=Forward Euler  ControllerParametersSource=internal  P=0  I=Rollrate.ki  D=0  UseFilter=on  N=100  TunerSelectOption=Transfer Function Based (PID Tuner App)  InitialConditionSource=internal  InitialConditionForIntegrator=0  InitialConditionForFilter=0  DifferentiatorICPrevScaledInput=0  ExternalReset=none  TrackingMode=off  Kt=1  LimitOutput=off  SatLimitsSource=internal  UpperSaturationLimit=inf  LowerSaturationLimit=-inf  LinearizeAsGain=on  AntiWindupMode=none  Kb=1  POutMin=[]  POutMax=[]  IOutMin=[]  IOutMax=[]  DOutMin=[]  DOutMax=[]  NOutMin=[]  NOutMax=[]  SumOutMin=[]  SumOutMax=[]  SaturationOutMin=[]  SaturationOutMax=[]  PParamMin=[]  PParamMax=[]  IParamMin=[]  IParamMax=[]  DParamMin=[]  DParamMax=[]  NParamMin=[]  NParamMax=[]  KbParamMin=[]  KbParamMax=[]  KtParamMin=[]  KtParamMax=[]  KbOutMin=[]  KbOutMax=[]  KtOutMin=[]  KtOutMax=[]  IntegratorOutMin=[]  IntegratorOutMax=[]  FilterOutMin=[]  FilterOutMax=[]  SumI1OutMin=[]  SumI1OutMax=[]  SumI2OutMin=[]  SumI2OutMax=[]  SumI3OutMin=[]  SumI3OutMax=[]  SumI4OutMin=[]  SumI4OutMax=[]  SumDOutMin=[]  SumDOutMax=[]  DifferentiatorOutMin=[]  DifferentiatorOutMax=[]  FilterDiffOutCoefMin=[]  FilterDiffOutCoefMax=[]  ReciprocalOutMin=[]  ReciprocalOutMax=[]  SumDenOutMin=[]  SumDenOutMax=[]  SumNumOutMin=[]  SumNumOutMax=[]  DivideOutMin=[]  DivideOutMax=[]  UdiffTsProdOutMin=[]  UdiffTsProdOutMax=[]  NTsProdOutMin=[]  NTsProdOutMax=[]  UintegralTsProdOutMin=[]  UintegralTsProdOutMax=[]  UngainTsProdOutMin=[]  UngainTsProdOutMax=[]  IntegratorContinuousStateAttributes=''  IntegratorStateMustResolveToSignalObject=off  IntegratorRTWStateStorageClass=Auto  FilterContinuousStateAttributes=''  FilterStateMustResolveToSignalObject=off  FilterRTWStateStorageClass=Auto  ParallelPVariant=InternalParameters  IdealPVariant=Disabled  IVariant=InternalParameters  DVariant=InternalParameters  IntegratorVariant=Continuous  SatVariant=Disabled  AWVariant=Passthrough  PCopyVariant=Disabled  TRVariant=Disabled  FdbkBlocksVariant=Forward  IdealPFdbkVariant=Disabled  SatFdbkVariant=Disabled  DerivativeFilterVariant=ContFilter  NVariant=InternalParameters  NCopyVariant=Disabled  FilterICVariant=InternalICsFilter  IntegratorICVariant=InternalICs  ExternalResetVariant=Disabled  TRSumVariant=Passthrough  SumFdbkVariant=Disabled  SumVariant=Sum_PID  TsampFilterVariant=InternalTs  TsampNgainVariant=Passthrough  TsampIntegralVariant=Passthrough  ExternalSaturationOutDataTypeStr=Inherit: Same as second input
  PID Controller2 : pid_lib/PID Controller  Controller=PID  Form=Parallel  TimeDomain=Continuous-time  UseExternalTs=off  SampleTime=-1  IntegratorMethod=Forward Euler  FilterMethod=Forward Euler  ControllerParametersSource=internal  P=Rollrate.kp  I=0  D=0  UseFilter=on  N=100  TunerSelectOption=Transfer Function Based (PID Tuner App)  InitialConditionSource=internal  InitialConditionForIntegrator=0  InitialConditionForFilter=0  DifferentiatorICPrevScaledInput=0  ExternalReset=none  TrackingMode=off  Kt=1  LimitOutput=off  SatLimitsSource=internal  UpperSaturationLimit=inf  LowerSaturationLimit=-inf  LinearizeAsGain=on  AntiWindupMode=none  Kb=1  POutMin=[]  POutMax=[]  IOutMin=[]  IOutMax=[]  DOutMin=[]  DOutMax=[]  NOutMin=[]  NOutMax=[]  SumOutMin=[]  SumOutMax=[]  SaturationOutMin=[]  SaturationOutMax=[]  PParamMin=[]  PParamMax=[]  IParamMin=[]  IParamMax=[]  DParamMin=[]  DParamMax=[]  NParamMin=[]  NParamMax=[]  KbParamMin=[]  KbParamMax=[]  KtParamMin=[]  KtParamMax=[]  KbOutMin=[]  KbOutMax=[]  KtOutMin=[]  KtOutMax=[]  IntegratorOutMin=[]  IntegratorOutMax=[]  FilterOutMin=[]  FilterOutMax=[]  SumI1OutMin=[]  SumI1OutMax=[]  SumI2OutMin=[]  SumI2OutMax=[]  SumI3OutMin=[]  SumI3OutMax=[]  SumI4OutMin=[]  SumI4OutMax=[]  SumDOutMin=[]  SumDOutMax=[]  DifferentiatorOutMin=[]  DifferentiatorOutMax=[]  FilterDiffOutCoefMin=[]  FilterDiffOutCoefMax=[]  ReciprocalOutMin=[]  ReciprocalOutMax=[]  SumDenOutMin=[]  SumDenOutMax=[]  SumNumOutMin=[]  SumNumOutMax=[]  DivideOutMin=[]  DivideOutMax=[]  UdiffTsProdOutMin=[]  UdiffTsProdOutMax=[]  NTsProdOutMin=[]  NTsProdOutMax=[]  UintegralTsProdOutMin=[]  UintegralTsProdOutMax=[]  UngainTsProdOutMin=[]  UngainTsProdOutMax=[]  IntegratorContinuousStateAttributes=''  IntegratorStateMustResolveToSignalObject=off  IntegratorRTWStateStorageClass=Auto  FilterContinuousStateAttributes=''  FilterStateMustResolveToSignalObject=off  FilterRTWStateStorageClass=Auto  ParallelPVariant=InternalParameters  IdealPVariant=Disabled  IVariant=InternalParameters  DVariant=InternalParameters  IntegratorVariant=Continuous  SatVariant=Disabled  AWVariant=Passthrough  PCopyVariant=Disabled  TRVariant=Disabled  FdbkBlocksVariant=Forward  IdealPFdbkVariant=Disabled  SatFdbkVariant=Disabled  DerivativeFilterVariant=ContFilter  NVariant=InternalParameters  NCopyVariant=Disabled  FilterICVariant=InternalICsFilter  IntegratorICVariant=InternalICs  ExternalResetVariant=Disabled  TRSumVariant=Passthrough  SumFdbkVariant=Disabled  SumVariant=Sum_PID  TsampFilterVariant=InternalTs  TsampNgainVariant=Passthrough  TsampIntegralVariant=Passthrough  ExternalSaturationOutDataTypeStr=Inherit: Same as second input
  Saturation : Saturate  UpperLimit=Rollrate.intupper  LowerLimit=Rollrate.intlower
  Scope : Scope  NumInputPorts=2
  Sum : Sum  Inputs=|++
  y : Outport
  wires:
  Saturation/1 -> Scope/1, Sum/2
  PID Controller1/1 -> Saturation/1, Scope/2
  Sum/1 -> y/1
  u/1 -> PID Controller2/1, PID Controller1/1
  PID Controller2/1 -> Sum/1

== matlab function CrazyClover_trajectory_tracking/moter map/gram->pwm2 ==
  data: x input; y2_invf output
function y2_invf = m2_map(x)
%#codegen

%    This function was generated by the Symbolic Math Toolbox version 8.6.
%    24-Aug-2022 00:51:31
if x > 0
    y2_invf = sqrt(x.*8.763965396891775e-7+1.033956593757182e-5).*2.282071995297151e+6-5.020028004430765e+3;
else
    x = abs(x);
    y2_invf = -(sqrt(x.*8.763965396891775e-7+1.033956593757182e-5).*2.282071995297151e+6-5.020028004430765e+3);
end

== matlab function CrazyClover_trajectory_tracking/moter map/gram->pwm3 ==
  data: x input; y3_invf output
function y3_invf = m3_map(x)
%#codegen

%    This function was generated by the Symbolic Math Toolbox version 8.6.
%    24-Aug-2022 00:51:31

if x > 0
    y3_invf = sqrt(x.*8.464410710967024e-7+1.206468234853723e-5).*2.362834305061159e+6-5.75446231128539e+3;
else
    x = abs(x);
    y3_invf = -(sqrt(x.*8.464410710967024e-7+1.206468234853723e-5).*2.362834305061159e+6-5.75446231128539e+3);
end

== matlab function CrazyClover_trajectory_tracking/moter map/gram->pwm4 ==
  data: x input; y4_invf output
function y4_invf = m4_map(x)
%#codegen

%    This function was generated by the Symbolic Math Toolbox version 8.6.
%    24-Aug-2022 00:51:31
if x > 0
    y4_invf = sqrt(x.*8.083914057959226e-7+1.102319411174238e-5).*2.474049062942287e+6-5.961111523577613e+3;
else
    x = abs(x);
    y4_invf = -(sqrt(x.*8.083914057959226e-7+1.102319411174238e-5).*2.474049062942287e+6-5.961111523577613e+3);
end

== matlab function CrazyClover_trajectory_tracking/State Feedback/Subsystem/MATLAB Function6 ==
  data: F input; Fz output; R input
function Fz = fcn(F, R)
e3 = [0;0;1];
u = dot(F, R*e3);

Fz = u;

== matlab function CrazyClover_trajectory_tracking/State Feedback/Subsystem/attitude translate ==
  data: roll input; R output; pitch input; yaw input
function R = fcn(roll, pitch, yaw)
% RPYから回転行列計算

R3 = [ cos(yaw) -sin(yaw) 0; sin(yaw) cos(yaw) 0; 0 0 1];              % ヨー角
R2 = [ cos(pitch) 0 sin(pitch); 0 1 0; -sin(pitch) 0 cos(pitch) ];     % ピッチ角
R1 = [ 1 0 0; 0 cos(roll) -sin(roll); 0 sin(roll) cos(roll)];          % ロール角

R = R3* R2 * R1;   % 回転行列（ボディー　-> ワールド）3

== matlab function CrazyClover_trajectory_tracking/Subsystem1/MATLAB Function2 ==
  data: RPY input; W input; Euler_angle_rate output
function Euler_angle_rate = fcn(RPY, W)
roll = RPY(1);
pitch = RPY(2);
yaw = RPY(3);
rollS = sin(roll); rollC = cos(roll);           
pitchS = sin(pitch); pitchC = cos(pitch);       


Euler_angle_rate = pinv([1 0 -pitchS;
     0 rollC  pitchC * rollS;
     0 -rollS pitchC * rollC]) * W;

== matlab function CrazyClover_trajectory_tracking/Subsystem1/Reference Trajectory ==
  data: ref_X output; ref_Vb output; ref_Accb output; ref_jarkb output; t input; T input; r input; ref_Yaw_Yawd output
function [ref_X, ref_Vb, ref_Accb, ref_jarkb, ref_Yaw_Yawd] = fcn(t,T,r)
% 軌道生成
w = 2 * pi/T;          % 角周波数

% 中心　半径　　
c = [0;0;0];

ref_X = c + r*[sin(w*t); cos(w*t); 0];
ref_Vb = r*[w*cos(w*t); -w*sin(w*t); 0];
ref_Accb = [-r*w^2*sin(w*t); -r*w^2*cos(w*t); 9.8];
ref_jarkb = r*[-w^3*cos(w*t); w^3*sin(w*t); 0];
ref_Yaw_Yawd = [0, 0]';

== matlab function CrazyClover_trajectory_tracking/Subsystem/MATLAB Function ==
  data: R input; Rd output; Wb input
function Rd = fcn(R, Wb)
wx = Wb(1);
wy = Wb(2);
wz = Wb(3);
Wb = [ 0    -wz   wy;
       wz    0   -wx;
      -wy    wx   0];
Rd = R * Wb;

== matlab function CrazyClover_trajectory_tracking/Subsystem1/Reference Attitude, Attitude rate  ==
  data: RPY output; Wbd output; t input; T input; r input
function [RPY, Wbd] = fcn(t,T,r)
% 軌道生成
w = 2 * pi/T;          % 角周波数

% 中心　半径　　
c = [0;0;0];

% Flat Outputから内部状態と入力揚力を計算
% 各軸の単位行列
e1 = [1; 0; 0];e2 = [0; 1; 0];e3 = [0; 0; 1];
% ドローンの質量　重力加速度
mQ = 0.027; g = 9.8;


x = c + r*[sin(w*t); cos(w*t); 0];         % 位置の軌道の位置
dx = r*[w*cos(w*t); -w*sin(w*t); 0];       % 速度の軌道
d2x = r*[-w^2*sin(w*t); -w^2*cos(w*t); 0]; % 加速度の軌道
d3x = r*[-w^3*cos(w*t); w^3*sin(w*t); 0];  % 加加速度の軌道
d4x = r*[w^4*sin(w*t); w^4*cos(w*t); 0];   % 加加加速度の軌道

alpha = 0;                                 
d_alpha = 0;                               
d2x(3) = d2x(3) + g;

pitch = atan( ( d2x(1)*cos(alpha) + d2x(2)*sin(alpha) ) / (d2x(3)));                                                        
roll = atan( ( d2x(1)*sin(alpha) - d2x(2)*cos(alpha) ) / sqrt( (d2x(3))^2 + ( d2x(1)*cos(alpha) + d2x(2)*sin(alpha) )^2));

rollS = sin(roll); rollC = cos(roll);           
pitchS = sin(pitch); pitchC = cos(pitch);       
yawS = sin(alpha); yawC = cos(alpha);           


% desired Roll rate
roll_rate_bunshi = d2x(3)^2 * ( d3x(1)*yawS - d3x(2)*yawC + d_alpha * (d2x(1)*yawC + d2x(2)*yawS) ) - d2x(3)*d3x(3)*(d2x(1)*yawS - d2x(2)*yawC) + (d2x(1)*yawC + d2x(2)*yawS)*(d_alpha*(d2x(1)^2 + d2x(2)^2) - d2x(1)*d3x(2) + d2x(2)*d3x(1));
roll_rate_bunbo = (d2x(1)^2 + d2x(2)^2 + d2x(3)^2) * sqrt(d2x(3)^2 + ( d2x(1)*yawC + d2x(2)*yawS )^2);
roll_rate = roll_rate_bunshi / roll_rate_bunbo;

% desired Pitch rate
pitch_rate_bunshi = d2x(3)*(d3x(1)*yawC + d3x(2)*yawS) - d3x(3)*(d2x(1)*yawC + d2x(2)*yawS) - d2x(3)*d_alpha*(d2x(1)*yawS + d2x(2)*yawC);
pitch_rate_bunbo = d2x(3)^2 + ( d2x(1)*yawC + d2x(2)*yawS )^2;
pitch_rate = pitch_rate_bunshi / pitch_rate_bunbo;

W = [1 0      -pitchS;
     0 rollC  pitchC * rollS;
     0 -rollS pitchC * rollC] * [roll_rate;pitch_rate;d_alpha];

RPY = [roll, pitch, alpha]';
Wbd = W;

== matlab function CrazyClover_trajectory_tracking/State Feedback/Subsystem/Calculate Attitude Error ==
  data: R input; ref_R input; eR output
function eR = fcn(R, ref_R)
transpose_R = R';
transpose_ref_R = ref_R';
tmp = -(transpose_ref_R*R - transpose_R*ref_R)/2;
eR = [tmp(3, 2), -tmp(3, 1), tmp(2, 1)];

== matlab function CrazyClover_trajectory_tracking/actuator/pwm -> gram ==
  data: m1_pwm input; m1 output; m2_pwm input; m3_pwm input; m4_pwm input; m2 output; m3 output; m4 output
function [m1, m2,m3, m4]= func(m1_pwm, m2_pwm, m3_pwm, m4_pwm)

% F [16bit] Wddb [16bit]

% m1_pwm = moter_in(1);
% m2_pwm = moter_in(2);
% m3_pwm = moter_in(3);
% m4_pwm = moter_in(4);
m1_map = [2.1910e-07 0.0022 0];
m2_map = [2.1910e-07 0.0022 0];
m3_map = [2.1161e-07 0.0024 0];
m4_map = [2.0210e-07 0.0024 0];
% m_avs = (m1_pwm + m2_pwm + m3_pwm + m4_pwm)/4;
% m1_pwm = m_avs;
% m2_pwm = m_avs;
% m3_pwm = m_avs;
% m4_pwm = m_avs;
if m1_pwm > 0
    m1 = m1_map * [m1_pwm^2;m1_pwm;1];
else
    m1 = -m1_map * [m1_pwm^2;-m1_pwm;1];
end
if m2_pwm > 0
    m2 = m2_map * [m2_pwm^2;m2_pwm;1];
else
    m2 = -m2_map * [m2_pwm^2;-m2_pwm;1];
end
if m3_pwm > 0
    m3 = m3_map * [m3_pwm^2;m3_pwm;1];
else
    m3 = -m3_map * [m3_pwm^2;-m3_pwm;1];
end
if m1_pwm > 0
    m4 = m4_map * [m4_pwm^2;m4_pwm;1];
else
    m4 = -m4_map * [m4_pwm^2;-m4_pwm;1];
end

== matlab function CrazyClover_trajectory_tracking/State Feedback/Subsystem/Calculate reference Attitude, Angular Velocity ==
  data: ref_R output; ref_W output; F input; ref_Accb input; ref_jark input; yaw input; yaw_dot input
function [ref_R, ref_W]= fcn(F, ref_Accb, ref_jark, yaw, yaw_dot)

% Flat Outputから内部状態と入力揚力を計算

m = 0.027;
% 各軸の単位行列
e1 = [1; 0; 0];e2 = [0; 1; 0];e3 = [0; 0; 1];
% ドローンの質量　重力加速度
mQ = 1; g = 9.8;

Xc = [cos(yaw) sin(yaw) 0]';          % よー角のベクトル　Rc(3)
Yc = [-sin(yaw) cos(yaw) 0]';
dXc = yaw_dot * Yc; % よー角のベクトルの微分
dYc = -yaw_dot * Xc; 
   
% 所望の姿勢を計算している
% 軌道の加速度のベクトル: b3 を計算
Zb = F / norm(F);   
%
Xb = cross(Yc, Zb)/norm(cross(Yc, Zb));
Yb = cross(Zb, Xb);
ref_R = [Xb Yb Zb] ;

% 加加速度ベクトルを計算
dfZb = ref_jark;
  
% 目標の姿勢のz軸方向のベクトルの微分を計算
dZb = dfZb/norm(F) - F * dot(F, dfZb)/norm(F)^3; % Zb_dot---------- dot(　fb1/norm(fb1) )

% 目標の姿勢のx軸方向のベクトルを計算
dnorm_Zb_Xc2 = norm(cross(dYc, Zb) + cross(Yc, dZb));
dXb = (cross(dYc, Zb) + cross(Yc, dZb))/dnorm_Zb_Xc2 - cross(Yc, Zb) * dot(cross(Yc, Zb),( cross(dYc, Zb) + cross(Yc, dZb)))/dnorm_Zb_Xc2^3;
   
% 目標の姿勢のy軸方向のベクトルを計算
dYb = cross(dZb, Xb) + cross(Zb, dXb) ;  %dot_b2 = dotb3とb1 の外積と　b3とdot_b1の外積　の和　--------- dot(cross(b3, b1))


wy = dot(Xb, ref_jark) / dot(Zb, ref_Accb);
wx = - dot(Yb, ref_jark) / dot(Zb, ref_Accb);
wz = (yaw_dot * dot(Xc, Xb) + wy * dot(Yc, Zb))/norm(cross(Yc, Zb));
ref_W = [wx wy wz];

== matlab function CrazyClover_trajectory_tracking/Subsystem/MATLAB Function2 ==
  data: W input; Euler_angle_rate output; RPY input
function Euler_angle_rate = fcn(W, RPY)
roll = RPY(1);
pitch = RPY(2);
yaw = RPY(3);
rollS = sin(roll); rollC = cos(roll);           
pitchS = sin(pitch); pitchC = cos(pitch);       


Euler_angle_rate = pinv([1 0 -pitchS;
     0 rollC  pitchC * rollS;
     0 -rollS pitchC * rollC]) * W;

== matlab function CrazyClover_trajectory_tracking/moter map/gram->pwm1 2 ==
  data: x input; y1_invf output
function y1_invf = m1_map(x)
%#codegen

%    This function was generated by the Symbolic Math Toolbox version 8.6.
%    24-Aug-2022 00:51:31
if x > 0
    y1_invf = sqrt(x.*8.309953163553529e-7+8.77420076969215e-6).*2.406752433662037e+6-4.951128620134714e+3;
else
    x = abs(x);
    y1_invf = -(sqrt(x.*8.309953163553529e-7+8.77420076969215e-6).*2.406752433662037e+6-4.951128620134714e+3);
end

== matlab function CrazyClover_trajectory_tracking/Subsystem/Dynamics1 ==
  data: F input; Pdd output; M input; Wb input; R input; Wdd output
function [Pdd, Wdd]  = fcn(F, M, Wb, R)
m = 500;
e3 = [0 0 1]';
g = 9.8;

% 各加速度計算（ボディー座標系）
Pdd = 9.8 * F*R*e3/m - g*e3;
I = [1 0 0;
     0 1 0;
     0 0 1]*10^(-3);
% 各加速度計算（ボディー座標系）
Wdd = pinv(I)*(M - cross(Wb, I * Wb));
